simulink model "pblm3_model"  (R2020b)
settings: Solver=VariableStepAuto  StartTime=0.0  StopTime=10.0  RelTol=1e-3
values from neighbouring files (symbols this model uses):
  a = -1    [MECH6313_HW4.m]
  b = 1    [MECH6313_HW4.m]
  K = place(A,B, [-1+j,-1-j])    [MECH6313_HW4.m]
libraries: cstblocks x1
settings Model: Creator=Jonas  LastModifiedBy=Jonas

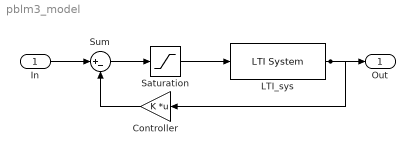
== system pblm3_model ==
  In : Inport
  Controller : Gain  Gain=K  Multiplication=Matrix(K*u)
  LTI_sys : cstblocks/LTI System  sys=lti_sys  IC=x0
  Saturation : Saturate  UpperLimit=b  LowerLimit=a
  Sum : Sum  Inputs=|+-
  Out : Outport
  wires:
  Saturation/1 -> LTI_sys/1
  Controller/1 -> Sum/2
  Sum/1 -> Saturation/1
  LTI_sys/1 -> Controller/1, Out/1
  In/1 -> Sum/1
